simulink model "Vending_machine"  (R2020b)
settings: Solver=VariableStepAuto  StartTime=0.0  StopTime=10.0  RelTol=1e-3
settings Model: Creator=ADMIN  LastModifiedBy=ADMIN

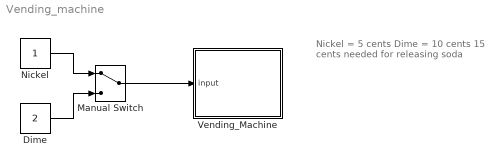
== system Vending_machine ==
  note: Nickel = 5 cents
      | Dime = 10 cents
      | 15 cents needed for releasing soda
  Dime : Constant  Value=2
  Manual Switch : ManualSwitch
  Nickel : Constant
  Vending_Machine : Stateflow chart  TreatAsAtomicUnit=on
  wires:
  Nickel/1 -> Manual Switch/1
  Dime/1 -> Manual Switch/2
  Manual Switch/1 -> Vending_Machine/1(input)

== stateflow chart Vending_machine/Vending_Machine ==
  settings: stateMachineType=MEALY_MACHINE
  state got_0
  state got_nickel
  state got_dime
  (default) -> got_0
  data: input input
